simulink model "file"  (R2023b)
settings: Solver=ode15s  StartTime=0.0  StopTime=7  MaxStep=1e-4  RelTol=1e-5
undefined symbols (not defined in the file or in its folder): dw_dt, ia_max, kamp, kdt, kff, ki, klim, kp, S_new2, T_regime, Td, Ts
settings Model: Creator=aniello  LastModifiedBy=aniello
settings SolverCC: ZeroCrossAlgorithm=Adaptive
settings DebuggingCC: AlgebraicLoopMsg=none  ArtificialAlgebraicLoopMsg=none  IgnoredZcDiagnostic=none

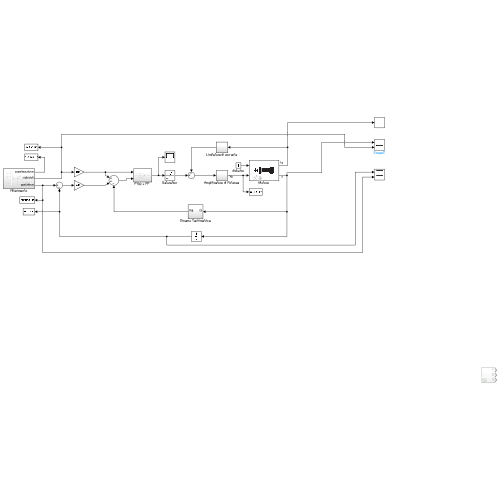
[thumbnail: Simulink's stored preview of the top-level diagram]
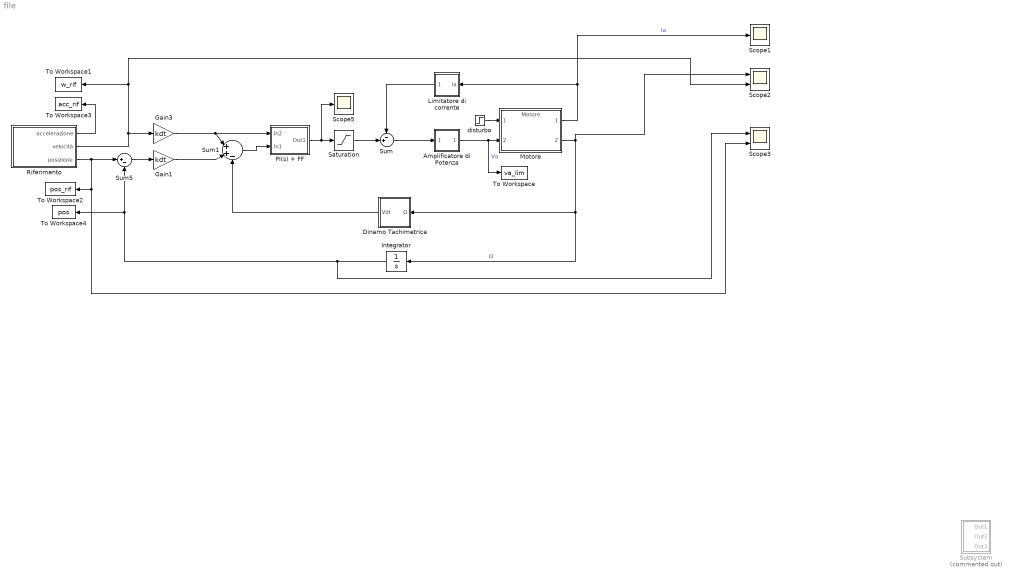
== system file ==
  Amplificatore di Potenza : Subsystem
  Dinamo Tachimetrica : Subsystem
  Gain1 : Gain  Gain=kdt
  Gain3 : Gain  Gain=kdt
  Integrator : Integrator
  Limitatore di corrente : Subsystem
  Motore : ModelReference  ModelNameDialog=Motore.slx  SimulationMode=Normal  ModelReferenceVersion=1.23
      mask Display: image('motore.jpg');
  "PI(s) + FF " : Subsystem
  Riferimento : Subsystem
  Saturation : Saturate  UpperLimit=5  LowerLimit=-5
  Scope1 : Scope
  Scope2 : Scope  NumInputPorts=2
  Scope3 : Scope  NumInputPorts=2
  Scope5 : Scope
  Subsystem : Subsystem  Commented=on
  Sum : Sum  Inputs=-+|
  Sum1 : Sum  Inputs=|++-
  Sum5 : Sum  Inputs=|+-
  To Workspace : ToWorkspace  VariableName=va_lim  SaveFormat=Timeseries  SampleTime=-1
  To Workspace1 : ToWorkspace  VariableName=w_rif  SaveFormat=Timeseries  SampleTime=-1
  To Workspace2 : ToWorkspace  VariableName=pos_rif  SaveFormat=Timeseries  SampleTime=-1
  To Workspace3 : ToWorkspace  VariableName=acc_rif  SaveFormat=Timeseries  SampleTime=-1
  To Workspace4 : ToWorkspace  VariableName=pos  SaveFormat=Timeseries  SampleTime=-1
  disturbo : Step  Time=3  After=0.057  SampleTime=0
  wires:
  Motore/1 -> Limitatore di corrente/1(Ia), Scope1/1  "Ia"
  Amplificatore di Potenza/1(Va) -> Motore/2, To Workspace/1  "Va"
  Sum/1 -> Amplificatore di Potenza/1(In1)
  Motore/2 -> Scope2/1, Integrator/1, Dinamo Tachimetrica/1(Ω)  "Ω"
  Limitatore di corrente/1(Out1) -> Sum/1
  Sum1/1 -> "PI(s) + FF "/2(In1)
  "PI(s) + FF "/1(Out1) -> Scope5/1, Saturation/1
  Riferimento/2(velocità) -> Scope2/2, To Workspace1/1, Gain3/1
  Dinamo Tachimetrica/1(Vdt) -> Sum1/3
  Riferimento/3(posizione) -> Scope3/2, To Workspace2/1, Sum5/1
  Integrator/1 -> To Workspace4/1, Sum5/2, Scope3/1
  Sum5/1 -> Gain1/1
  Gain3/1 -> Sum1/1, "PI(s) + FF "/1(In2)
  Saturation/1 -> Sum/2
  Gain1/1 -> Sum1/2
  Riferimento/1(accelerazione) -> To Workspace3/1
  disturbo/1 -> Motore/1

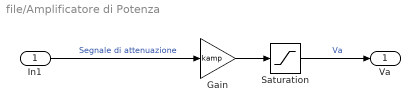
== system file/Amplificatore di Potenza ==
  In1 : Inport
  Gain : Gain  Gain=kamp
  Saturation : Saturate  UpperLimit=40.32  LowerLimit=-40.32
  Va : Outport
  wires:
  In1/1 -> Gain/1  "Segnale di attenuazione"
  Saturation/1 -> Va/1  "Va"
  Gain/1 -> Saturation/1

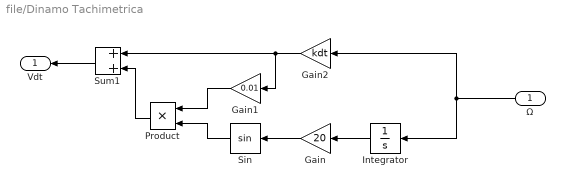
== system file/Dinamo Tachimetrica ==
  Ω : Inport
  Gain : Gain  Gain=20
  Gain1 : Gain  Gain=0.01
  Gain2 : Gain  Gain=kdt
  Integrator : Integrator
  Product : Product
  Sin : Trigonometry
  Sum1 : Sum
  Vdt : Outport
  wires:
  Sin/1 -> Product/2
  Ω/1 -> Integrator/1, Gain2/1
  Integrator/1 -> Gain/1
  Gain/1 -> Sin/1
  Gain2/1 -> Gain1/1, Sum1/1
  Product/1 -> Sum1/2
  Sum1/1 -> Vdt/1
  Gain1/1 -> Product/1

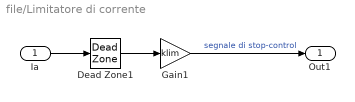
== system file/Limitatore di corrente ==
  Ia : Inport
  Dead Zone1 : DeadZone  LowerValue=-ia_max  UpperValue=ia_max
  Gain1 : Gain  Gain=klim
  Out1 : Outport
  wires:
  Dead Zone1/1 -> Gain1/1
  Ia/1 -> Dead Zone1/1
  Gain1/1 -> Out1/1  "segnale di stop-control"

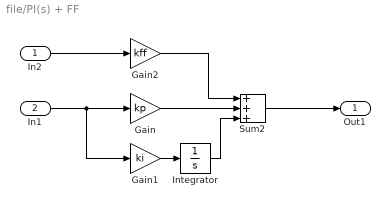
== system file/PI(s) + FF  ==
  In2 : Inport
  In1 : Inport  Port=2
  Gain : Gain  Gain=kp
  Gain1 : Gain  Gain=ki
  Gain2 : Gain  Gain=kff
  Integrator : Integrator  LimitOutput=on  UpperSaturationLimit=S_new2  LowerSaturationLimit=-S_new2
  Sum2 : Sum  Inputs=+++
  Out1 : Outport
  wires:
  Sum2/1 -> Out1/1
  In1/1 -> Gain1/1, Gain/1
  Gain1/1 -> Integrator/1
  Gain/1 -> Sum2/2
  Integrator/1 -> Sum2/3
  In2/1 -> Gain2/1
  Gain2/1 -> Sum2/1

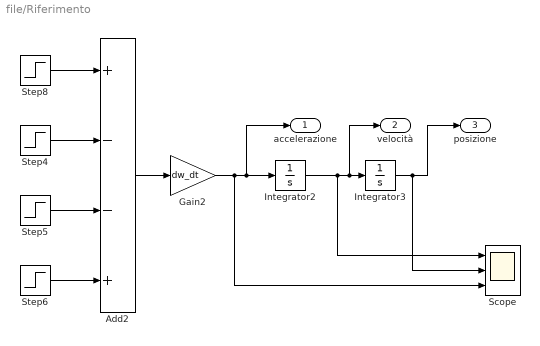
== system file/Riferimento ==
  Add2 : Sum  Inputs=+--+
  Gain2 : Gain  Gain=dw_dt
  Integrator2 : Integrator  UpperSaturationLimit=0.3707  LowerSaturationLimit=-0.3707
  Integrator3 : Integrator  UpperSaturationLimit=0.3707  LowerSaturationLimit=-0.3707
  Scope : Scope  NumInputPorts=3
  Step4 : Step  Time=Ts+0.2  SampleTime=0
  Step5 : Step  Time=Ts+T_regime+0.2  SampleTime=0
  Step6 : Step  Time=Ts+T_regime+Td+0.2  SampleTime=0
  Step8 : Step  Time=0.2  SampleTime=0
  accelerazione : Outport
  velocità : Outport  Port=2
  posizione : Outport  Port=3
  wires:
  Step6/1 -> Add2/4
  Integrator2/1 -> Scope/1, velocità/1, Integrator3/1
  Step5/1 -> Add2/3
  Step8/1 -> Add2/1
  Step4/1 -> Add2/2
  Integrator3/1 -> Scope/2, posizione/1
  Add2/1 -> Gain2/1
  Gain2/1 -> Scope/3, accelerazione/1, Integrator2/1

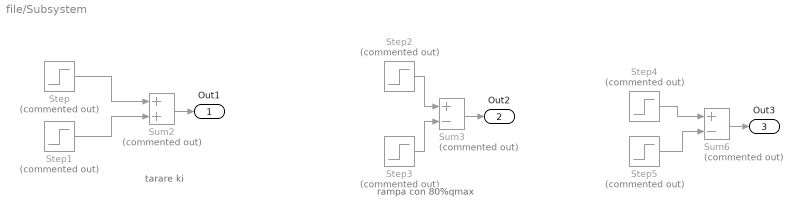
== system file/Subsystem ==
  note: tarare ki
  note: rampa con 80%qmax
  Step : Step  Commented=on  Time=0.1  After=3.4423  SampleTime=0
  Step1 : Step  Commented=on  Time=4  After=0.01575  SampleTime=0
  Step2 : Step  Commented=on  Time=0  SampleTime=0
  Step3 : Step  Commented=on  Time=1.562  SampleTime=0
  Step4 : Step  Commented=on  Time=3  After=0.2  SampleTime=0
  Step5 : Step  Commented=on  Time=3.05  After=0.2  SampleTime=0
  Sum2 : Sum  Commented=on
  Sum3 : Sum  Commented=on  Inputs=+-
  Sum6 : Sum  Commented=on  Inputs=+-
  Out1 : Outport
  Out2 : Outport  Port=2
  Out3 : Outport  Port=3
  wires:
  Sum2/1 -> Out1/1
  Step1/1 -> Sum2/2
  Sum6/1 -> Out3/1
  Step2/1 -> Sum3/1
  Step5/1 -> Sum6/2
  Step/1 -> Sum2/1
  Sum3/1 -> Out2/1
  Step3/1 -> Sum3/2
  Step4/1 -> Sum6/1
